simulink model "test_atrias"  (R2014b)
settings: Solver=FixedStepDiscrete  StartTime=0.0  StopTime=inf  FixedStep=0.001  RelTol=1e-3
StartFcn:
  | tg.sampletime = correctedSampleTime;
libraries: xpcethercatlib x62, simulink x41, slrtlib x12
settings Model: xpc_rtwmakecfg_data=_xpcethercatlib_  SimulationMode=external  BufferReuse=off  Creator=drl  LastModifiedBy=drl
settings SolverCC: EnableConcurrentExecution=on  ConcurrentTasks=on
settings OptimizationCC: BlockReduction=off  OptimizeBlockIOStorage=off  BufferReuse=off  GlobalBufferReuse=off  ExpressionFolding=off  LocalBlockOutputs=off
settings HardwareCC: ProdIntDivRoundTo=Zero  ProdEndianess=LittleEndian  ProdLongLongMode=on  ProdHWDeviceType=Generic->32-bit x86 compatible
settings RTWCC: SystemTargetFile=slrt.tlc  TemplateMakefile=slrt_default_tmf  Description=Simulink Real-Time  ProcessScript=slrt_make_rtw_hook  RTWCompilerOptimization=On
settings SimulinkRealTimeCC: GeneratePreprocessorConditionals=Disable all  EnableShiftOperators=on

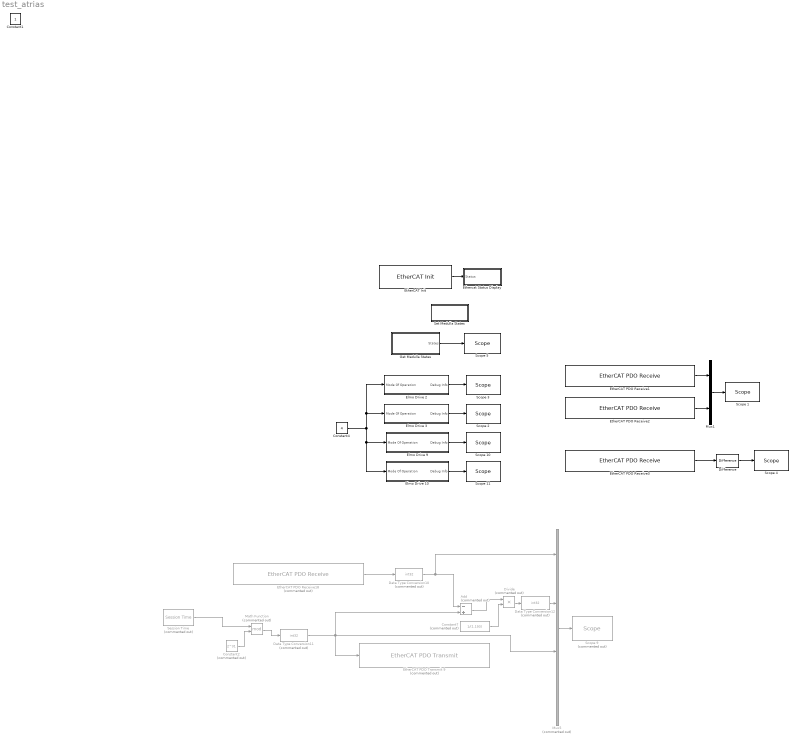
== system test_atrias ==
  Add : Sum  Commented=on  Inputs=-+
  Constant2 : Constant  Commented=on  Value=2^31
  Constant4 : Constant  Value=4  OutDataTypeStr=Inherit: Inherit via back propagation  SampleTime=-1
  Constant7 : Constant  Commented=on  Value=1/(1.193)
  Data Type Conversion10 : DataTypeConversion  Commented=on  OutDataTypeStr=int32
  Data Type Conversion11 : DataTypeConversion  Commented=on  OutDataTypeStr=int32
  Data Type Conversion12 : DataTypeConversion  Commented=on  OutDataTypeStr=int32
  Difference : simulink/Discrete/Difference  ICPrevInput=0.0  InputProcessing=Inherited  OutMin=[]  OutMax=[]  OutDataType=fixdt(1, 16)  OutScaling=2^-10  DoSatur=off
  Divide : Product  Commented=on  Inputs=**
  Elmo Drive 10 : Subsystem
  Elmo Drive 2 : Subsystem
  Elmo Drive 3 : Subsystem
  Elmo Drive 9 : Subsystem
  EtherCAT Init : xpcethercatlib/EtherCAT Init   Priority=0  config_file=8medullas4elmos_eni.xml  device_id=0  pci_bus=2  pci_slot=0  enaDebug=off  enaDC=on  errLink=off  masterDbg=off  stateChgDbg=off  baseClock=off  masterCfg=off  logFile='c:\dbglog.txt'  sample_time=0.001000
  EtherCAT PDO Receive1 : xpcethercatlib/EtherCAT PDO Receive  Priority=2  sig_name=Box 1 (ATRIAS 2.1 Hip (Medulla 1.5)).Hip Encoder.Encoder  sig_offset=504  sig_type=uint32  type_size=32  sig_dim=1  device_id=0  sample_time=0.001000
  EtherCAT PDO Receive18 : xpcethercatlib/EtherCAT PDO Receive  Priority=2  Commented=on  sig_name=Box 6 (ATRIAS 2.1 Leg (Medulla 1.5)).Motor Encoder.Motor Encoder  sig_offset=1648  sig_type=uint32  type_size=32  sig_dim=1  device_id=0  sample_time=0.001000
  EtherCAT PDO Receive2 : xpcethercatlib/EtherCAT PDO Receive  Priority=2  sig_name=Box 12 (ATRIAS 2.1 Boom (Medulla 1.5)).X Encoder.Encoder  sig_offset=2752  sig_type=uint32  type_size=32  sig_dim=1  device_id=0  sample_time=0.001000
  EtherCAT PDO Receive3 : xpcethercatlib/EtherCAT PDO Receive  Priority=2  sig_name=Box 1 (ATRIAS 2.1 Hip (Medulla 1.5)).uController Status.Counter  sig_offset=480  sig_type=uint8  type_size=8  sig_dim=1  device_id=0  sample_time=0.001000
  EtherCAT PDO Transmit 9 : xpcethercatlib/EtherCAT PDO Transmit   Priority=3  Commented=on  sig_name=Box 6 (ATRIAS 2.1 Leg (Medulla 1.5)).uControllerInput.Motor Current  sig_offset=1616  sig_type=int32  type_size=32  sig_dim=1  device_id=0  sample_time=0.001000
  Ethercat Status Display : Subsystem
  Get Medulla States : Subsystem
  Math Function : Math  Commented=on  Operator=mod  SaturateOnIntegerOverflow=on
  Mux1 : Mux  Inputs=2
  Mux5 : Mux  Commented=on
  Scope 1 : slrtlib/Displays and Logging/Scope   scopeno=8  scopetype=Target  autostart=on  viewmode=Graphical sliding  formatstr='%f'  grid=on  ylimits=[0,0]  nosamples=10000  noprepostsamples=0  interleave=1  triggermode=FreeRun  triggersignal=1  trigsignalfromport=off  triggerlevel=0.0  triggerslope=Either  triggerscope=1  triggersample=0  filename=data.dat  mode=Lazy  writesize=512  autorestart=off  dynamicfilemode=off  maxwritefilesize=512*1024^2
  Scope 10 : slrtlib/Displays and Logging/Scope   scopeno=3  scopetype=Target  autostart=on  viewmode=Numerical  formatstr='%f'  grid=on  ylimits=[0,0]  nosamples=10000  noprepostsamples=0  interleave=1  triggermode=FreeRun  triggersignal=1  trigsignalfromport=off  triggerlevel=0.0  triggerslope=Either  triggerscope=1  triggersample=0  filename=data.dat  mode=Lazy  writesize=512  autorestart=off  dynamicfilemode=off  maxwritefilesize=512*1024^2
  Scope 11 : slrtlib/Displays and Logging/Scope   scopeno=4  scopetype=Target  autostart=on  viewmode=Numerical  formatstr='%f'  grid=on  ylimits=[0,0]  nosamples=10000  noprepostsamples=0  interleave=1  triggermode=FreeRun  triggersignal=1  trigsignalfromport=off  triggerlevel=0.0  triggerslope=Either  triggerscope=1  triggersample=0  filename=data.dat  mode=Lazy  writesize=512  autorestart=off  dynamicfilemode=off  maxwritefilesize=512*1024^2
  Scope 2 : slrtlib/Displays and Logging/Scope   scopeno=2  scopetype=Target  autostart=on  viewmode=Numerical  formatstr='%f'  grid=on  ylimits=[0,0]  nosamples=10000  noprepostsamples=0  interleave=1  triggermode=FreeRun  triggersignal=1  trigsignalfromport=off  triggerlevel=0.0  triggerslope=Either  triggerscope=1  triggersample=0  filename=data.dat  mode=Lazy  writesize=512  autorestart=off  dynamicfilemode=off  maxwritefilesize=512*1024^2
  Scope 3 : slrtlib/Displays and Logging/Scope   scopeno=1  scopetype=Target  autostart=on  viewmode=Numerical  formatstr='%f'  grid=on  ylimits=[0,0]  nosamples=10000  noprepostsamples=0  interleave=1  triggermode=FreeRun  triggersignal=1  trigsignalfromport=off  triggerlevel=0.0  triggerslope=Either  triggerscope=1  triggersample=0  filename=data.dat  mode=Lazy  writesize=512  autorestart=off  dynamicfilemode=off  maxwritefilesize=512*1024^2
  Scope 4 : slrtlib/Displays and Logging/Scope   scopeno=9  scopetype=Target  autostart=on  viewmode=Graphical sliding  formatstr='%f'  grid=on  ylimits=[0,0]  nosamples=10000  noprepostsamples=0  interleave=1  triggermode=FreeRun  triggersignal=1  trigsignalfromport=off  triggerlevel=0.0  triggerslope=Either  triggerscope=1  triggersample=0  filename=data.dat  mode=Lazy  writesize=512  autorestart=off  dynamicfilemode=off  maxwritefilesize=512*1024^2
  Scope 5 : slrtlib/Displays and Logging/Scope   scopeno=7  scopetype=Target  autostart=on  viewmode=Numerical  formatstr='%f'  grid=on  ylimits=[0,0]  nosamples=100  noprepostsamples=0  interleave=1  triggermode=FreeRun  triggersignal=1  trigsignalfromport=off  triggerlevel=0.0  triggerslope=Either  triggerscope=1  triggersample=0  filename=data.dat  mode=Lazy  writesize=512  autorestart=off  dynamicfilemode=off  maxwritefilesize=512*1024^2
  Scope 9 : slrtlib/Displays and Logging/Scope   Commented=on  scopeno=10  scopetype=Target  autostart=on  viewmode=Numerical  formatstr='%f'  grid=on  ylimits=[0,0]  nosamples=100  noprepostsamples=0  interleave=1  triggermode=FreeRun  triggersignal=1  trigsignalfromport=off  triggerlevel=0.0  triggerslope=Either  triggerscope=1  triggersample=0  filename=data.dat  mode=Lazy  writesize=512  autorestart=off  dynamicfilemode=off  maxwritefilesize=512*1024^2
  "Session Time " : slrtlib/Target Management/Target Information/Session Time   Commented=on  ts=0.001
  Set Medulla States : Subsystem
  Constant1 : Constant  IOType=siggen
  wires:
  EtherCAT Init/1 -> Ethercat Status Display/1(Status)
  EtherCAT PDO Receive18/1 -> Data Type Conversion10/1
  Mux5/1 -> Scope 9/1
  Data Type Conversion10/1 -> Mux5/1, Add/1
  Constant2/1 -> Math Function/2
  Math Function/1 -> Data Type Conversion11/1
  Data Type Conversion11/1 -> EtherCAT PDO Transmit 9/1, Mux5/3, Add/2
  "Session Time "/1 -> Math Function/1
  Constant7/1 -> Divide/2
  Add/1 -> Divide/1
  Data Type Conversion12/1 -> Mux5/2
  Divide/1 -> Data Type Conversion12/1
  Elmo Drive 3/1(Debug Info) -> Scope 2/1
  Elmo Drive 2/1(Debug Info) -> Scope 3/1
  Elmo Drive 9/1(Debug Info) -> Scope 10/1
  Elmo Drive 10/1(Debug Info) -> Scope 11/1
  Constant4/1 -> Elmo Drive 9/1(Mode Of Operation), Elmo Drive 10/1(Mode Of Operation), Elmo Drive 3/1(Mode Of Operation), Elmo Drive 2/1(Mode Of Operation)
  Get Medulla States/1(States) -> Scope 5/1
  EtherCAT PDO Receive2/1 -> Mux1/2
  EtherCAT PDO Receive1/1 -> Mux1/1
  Mux1/1 -> Scope 1/1
  EtherCAT PDO Receive3/1 -> Difference/1
  Difference/1 -> Scope 4/1

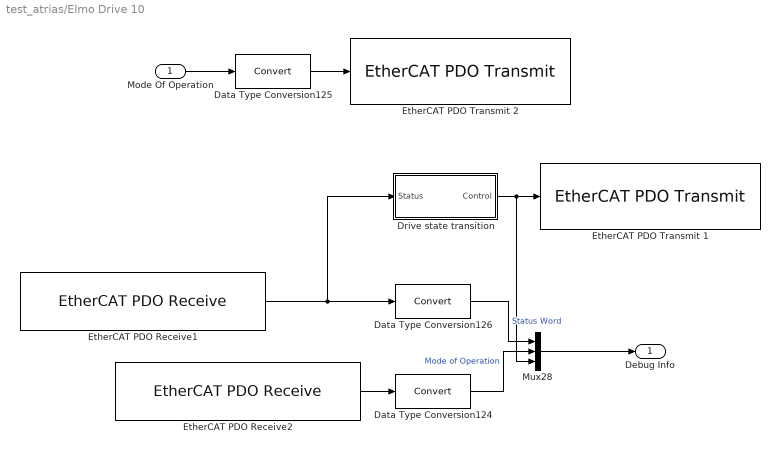
== system test_atrias/Elmo Drive 10 ==
  Mode Of Operation : Inport
  Data Type Conversion124 : DataTypeConversion
  Data Type Conversion125 : DataTypeConversion
  Data Type Conversion126 : DataTypeConversion
  Drive state transition : Subsystem
  EtherCAT PDO Receive1 : xpcethercatlib/EtherCAT PDO Receive  Priority=2  sig_name=Drive 10 (Elmo Drive).Inputs.Status word  sig_offset=3296  sig_type=uint16  type_size=16  sig_dim=1  device_id=0  sample_time=0.001000
  EtherCAT PDO Receive2 : xpcethercatlib/EtherCAT PDO Receive  Priority=2  sig_name=Drive 10 (Elmo Drive).Inputs.Mode of operation display  sig_offset=3312  sig_type=int8  type_size=8  sig_dim=1  device_id=0  sample_time=0.001000
  EtherCAT PDO Transmit 1 : xpcethercatlib/EtherCAT PDO Transmit   Priority=3  sig_name=Drive 10 (Elmo Drive).Outputs.Control word  sig_offset=3264  sig_type=uint16  type_size=16  sig_dim=1  device_id=0  sample_time=0.001000
  EtherCAT PDO Transmit 2 : xpcethercatlib/EtherCAT PDO Transmit   Priority=3  sig_name=Drive 10 (Elmo Drive).Outputs.Mode of operation  sig_offset=3280  sig_type=int8  type_size=8  sig_dim=1  device_id=0  sample_time=0.001000
  Mux28 : Mux  Inputs=3
  Debug Info : Outport
  wires:
  EtherCAT PDO Receive1/1 -> Drive state transition/1(Status), Data Type Conversion126/1
  EtherCAT PDO Receive2/1 -> Data Type Conversion124/1
  Mux28/1 -> Debug Info/1
  Data Type Conversion126/1 -> Mux28/1  "Status Word"
  Data Type Conversion124/1 -> Mux28/2  "Mode of Operation"
  Mode Of Operation/1 -> Data Type Conversion125/1
  Drive state transition/1(Control) -> Mux28/3, EtherCAT PDO Transmit 1/1
  Data Type Conversion125/1 -> EtherCAT PDO Transmit 2/1

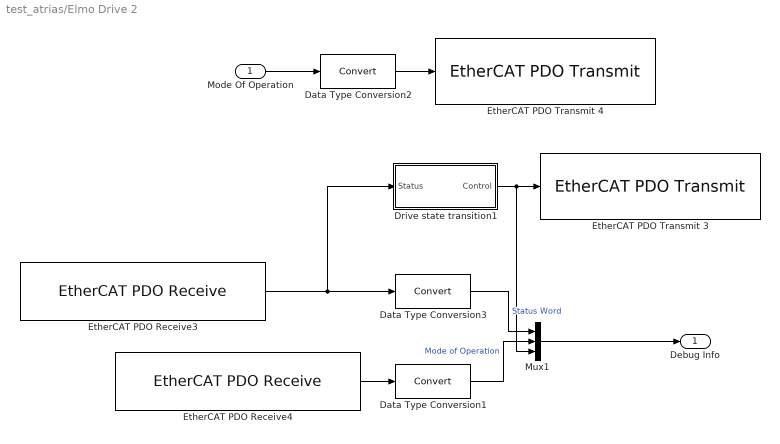
== system test_atrias/Elmo Drive 2 ==
  Mode Of Operation : Inport
  Data Type Conversion1 : DataTypeConversion
  Data Type Conversion2 : DataTypeConversion
  Data Type Conversion3 : DataTypeConversion
  Drive state transition1 : Subsystem
  EtherCAT PDO Receive3 : xpcethercatlib/EtherCAT PDO Receive  Priority=2  sig_name=Drive 2 (Elmo Drive).Inputs.Status word  sig_offset=3056  sig_type=uint16  type_size=16  sig_dim=1  device_id=0  sample_time=0.001000
  EtherCAT PDO Receive4 : xpcethercatlib/EtherCAT PDO Receive  Priority=2  sig_name=Drive 2 (Elmo Drive).Inputs.Mode of operation display  sig_offset=3072  sig_type=int8  type_size=8  sig_dim=1  device_id=0  sample_time=0.001000
  EtherCAT PDO Transmit 3 : xpcethercatlib/EtherCAT PDO Transmit   Priority=3  sig_name=Drive 2 (Elmo Drive).Outputs.Control word  sig_offset=3024  sig_type=uint16  type_size=16  sig_dim=1  device_id=0  sample_time=0.001000
  EtherCAT PDO Transmit 4 : xpcethercatlib/EtherCAT PDO Transmit   Priority=3  sig_name=Drive 2 (Elmo Drive).Outputs.Mode of operation  sig_offset=3040  sig_type=int8  type_size=8  sig_dim=1  device_id=0  sample_time=0.001000
  Mux1 : Mux  Inputs=3
  Debug Info : Outport
  wires:
  EtherCAT PDO Receive3/1 -> Drive state transition1/1(Status), Data Type Conversion3/1
  EtherCAT PDO Receive4/1 -> Data Type Conversion1/1
  Mux1/1 -> Debug Info/1
  Data Type Conversion3/1 -> Mux1/1  "Status Word"
  Data Type Conversion1/1 -> Mux1/2  "Mode of Operation"
  Mode Of Operation/1 -> Data Type Conversion2/1
  Drive state transition1/1(Control) -> Mux1/3, EtherCAT PDO Transmit 3/1
  Data Type Conversion2/1 -> EtherCAT PDO Transmit 4/1

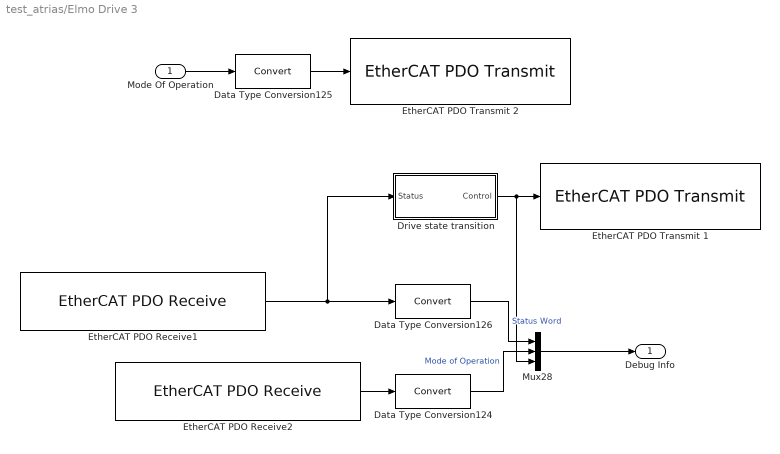
== system test_atrias/Elmo Drive 3 ==
  Mode Of Operation : Inport
  Data Type Conversion124 : DataTypeConversion
  Data Type Conversion125 : DataTypeConversion
  Data Type Conversion126 : DataTypeConversion
  Drive state transition : Subsystem
  EtherCAT PDO Receive1 : xpcethercatlib/EtherCAT PDO Receive  Priority=2  sig_name=Drive 3 (Elmo Drive).Inputs.Status word  sig_offset=3136  sig_type=uint16  type_size=16  sig_dim=1  device_id=0  sample_time=0.001000
  EtherCAT PDO Receive2 : xpcethercatlib/EtherCAT PDO Receive  Priority=2  sig_name=Drive 3 (Elmo Drive).Inputs.Mode of operation display  sig_offset=3152  sig_type=int8  type_size=8  sig_dim=1  device_id=0  sample_time=0.001000
  EtherCAT PDO Transmit 1 : xpcethercatlib/EtherCAT PDO Transmit   Priority=3  sig_name=Drive 3 (Elmo Drive).Outputs.Control word  sig_offset=3104  sig_type=uint16  type_size=16  sig_dim=1  device_id=0  sample_time=0.001000
  EtherCAT PDO Transmit 2 : xpcethercatlib/EtherCAT PDO Transmit   Priority=3  sig_name=Drive 3 (Elmo Drive).Outputs.Mode of operation  sig_offset=3120  sig_type=int8  type_size=8  sig_dim=1  device_id=0  sample_time=0.001000
  Mux28 : Mux  Inputs=3
  Debug Info : Outport
  wires:
  EtherCAT PDO Receive1/1 -> Drive state transition/1(Status), Data Type Conversion126/1
  EtherCAT PDO Receive2/1 -> Data Type Conversion124/1
  Mux28/1 -> Debug Info/1
  Data Type Conversion126/1 -> Mux28/1  "Status Word"
  Data Type Conversion124/1 -> Mux28/2  "Mode of Operation"
  Mode Of Operation/1 -> Data Type Conversion125/1
  Drive state transition/1(Control) -> Mux28/3, EtherCAT PDO Transmit 1/1
  Data Type Conversion125/1 -> EtherCAT PDO Transmit 2/1

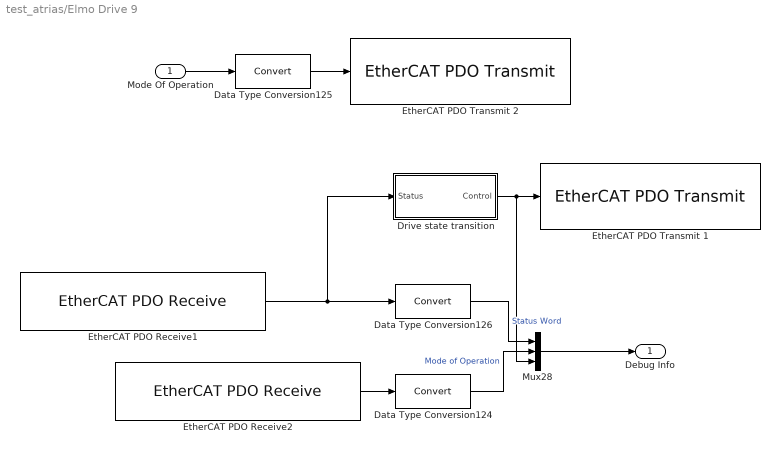
== system test_atrias/Elmo Drive 9 ==
  Mode Of Operation : Inport
  Data Type Conversion124 : DataTypeConversion
  Data Type Conversion125 : DataTypeConversion
  Data Type Conversion126 : DataTypeConversion
  Drive state transition : Subsystem
  EtherCAT PDO Receive1 : xpcethercatlib/EtherCAT PDO Receive  Priority=2  sig_name=Drive 9 (Elmo Drive).Inputs.Status word  sig_offset=3216  sig_type=uint16  type_size=16  sig_dim=1  device_id=0  sample_time=0.001000
  EtherCAT PDO Receive2 : xpcethercatlib/EtherCAT PDO Receive  Priority=2  sig_name=Drive 9 (Elmo Drive).Inputs.Mode of operation display  sig_offset=3232  sig_type=int8  type_size=8  sig_dim=1  device_id=0  sample_time=0.001000
  EtherCAT PDO Transmit 1 : xpcethercatlib/EtherCAT PDO Transmit   Priority=3  sig_name=Drive 9 (Elmo Drive).Outputs.Control word  sig_offset=3184  sig_type=uint16  type_size=16  sig_dim=1  device_id=0  sample_time=0.001000
  EtherCAT PDO Transmit 2 : xpcethercatlib/EtherCAT PDO Transmit   Priority=3  sig_name=Drive 9 (Elmo Drive).Outputs.Mode of operation  sig_offset=3200  sig_type=int8  type_size=8  sig_dim=1  device_id=0  sample_time=0.001000
  Mux28 : Mux  Inputs=3
  Debug Info : Outport
  wires:
  Data Type Conversion125/1 -> EtherCAT PDO Transmit 2/1
  Drive state transition/1(Control) -> EtherCAT PDO Transmit 1/1, Mux28/3
  Mode Of Operation/1 -> Data Type Conversion125/1
  Data Type Conversion124/1 -> Mux28/2  "Mode of Operation"
  Data Type Conversion126/1 -> Mux28/1  "Status Word"
  Mux28/1 -> Debug Info/1
  EtherCAT PDO Receive2/1 -> Data Type Conversion124/1
  EtherCAT PDO Receive1/1 -> Data Type Conversion126/1, Drive state transition/1(Status)

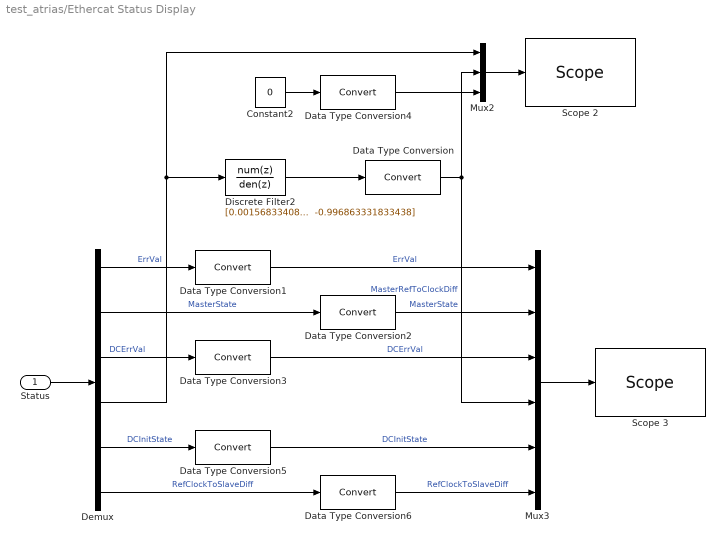
== system test_atrias/Ethercat Status Display ==
  Status : Inport
  Constant2 : Constant  Value=0  OutDataTypeStr=Inherit: Inherit via back propagation  SampleTime=-1
  Data Type Conversion{,1..6} (7 alike) : DataTypeConversion
  Demux : Demux  Outputs=6
  Discrete Filter2 : DiscreteFilter  Numerator="[0.001568334083281   0.001568334083281]"  Denominator="[1.000000000000000  -0.996863331833438]"  a0EqualsOne=on
  Mux2 : Mux  Inputs=3
  Mux3 : Mux  Inputs=6
  Scope 2 : slrtlib/Displays and Logging/Scope   scopeno=5  scopetype=Target  autostart=on  viewmode=Graphical rolling  formatstr='%f'  grid=on  ylimits=[0,0]  nosamples=10000  noprepostsamples=0  interleave=1  triggermode=FreeRun  triggersignal=1  trigsignalfromport=off  triggerlevel=0.0  triggerslope=Either  triggerscope=1  triggersample=0  filename=data.dat  mode=Lazy  writesize=512  autorestart=off  dynamicfilemode=off  maxwritefilesize=512*1024^2
  Scope 3 : slrtlib/Displays and Logging/Scope   scopeno=6  scopetype=Target  autostart=on  viewmode=Numerical  formatstr='%15.6f'  grid=on  ylimits=[0,0]  nosamples=100  noprepostsamples=0  interleave=1  triggermode=FreeRun  triggersignal=1  trigsignalfromport=off  triggerlevel=0.0  triggerslope=Either  triggerscope=1  triggersample=0  filename=data.dat  mode=Lazy  writesize=512  autorestart=off  dynamicfilemode=off  maxwritefilesize=512*1024^2
  wires:
  Status/1 -> Demux/1
  Demux/4 -> Discrete Filter2/1, Mux2/1
  Discrete Filter2/1 -> Data Type Conversion/1
  Mux2/1 -> Scope 2/1
  Constant2/1 -> Data Type Conversion4/1
  Data Type Conversion4/1 -> Mux2/3
  Mux3/1 -> Scope 3/1
  Data Type Conversion/1 -> Mux3/4, Mux2/2  "MasterRefToClockDiff"
  Data Type Conversion1/1 -> Mux3/1  "ErrVal"
  Data Type Conversion2/1 -> Mux3/2  "MasterState"
  Data Type Conversion3/1 -> Mux3/3  "DCErrVal"
  Data Type Conversion5/1 -> Mux3/5  "DCInitState"
  Data Type Conversion6/1 -> Mux3/6  "RefClockToSlaveDiff"
  Demux/1 -> Data Type Conversion1/1  "ErrVal"
  Demux/2 -> Data Type Conversion2/1  "MasterState"
  Demux/3 -> Data Type Conversion3/1  "DCErrVal"
  Demux/5 -> Data Type Conversion5/1  "DCInitState"
  Demux/6 -> Data Type Conversion6/1  "RefClockToSlaveDiff"

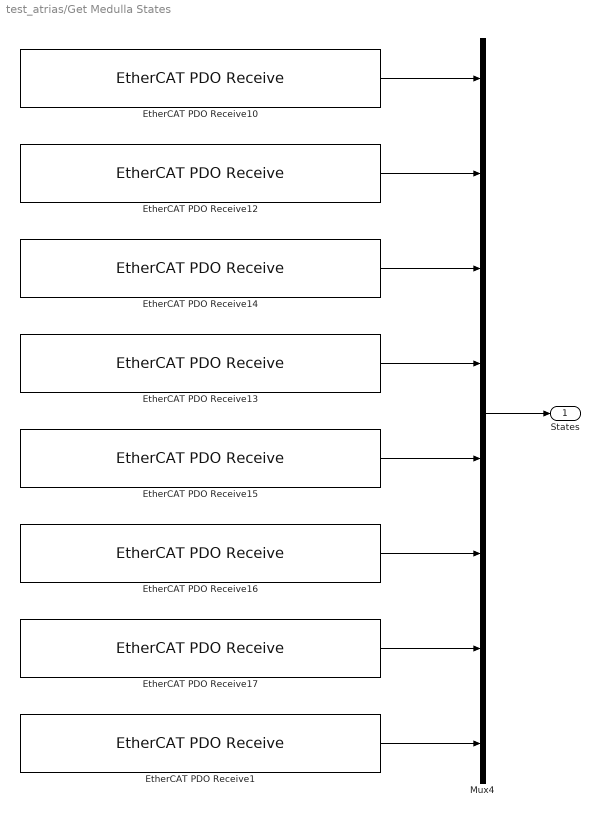
== system test_atrias/Get Medulla States ==
  EtherCAT PDO Receive1 : xpcethercatlib/EtherCAT PDO Receive  Priority=2  sig_name=Box 12 (ATRIAS 2.1 Boom (Medulla 1.5)).uController Status.State  sig_offset=2728  sig_type=uint8  type_size=8  sig_dim=1  device_id=0  sample_time=0.001000
  EtherCAT PDO Receive10 : xpcethercatlib/EtherCAT PDO Receive  Priority=2  sig_name=Box 1 (ATRIAS 2.1 Hip (Medulla 1.5)).uController Status.State  sig_offset=472  sig_type=uint8  type_size=8  sig_dim=1  device_id=0  sample_time=0.001000
  EtherCAT PDO Receive12 : xpcethercatlib/EtherCAT PDO Receive  Priority=2  sig_name=Box 4 (ATRIAS 2.1 IMU (Medulla 1.5)).uController Status.State  sig_offset=720  sig_type=uint8  type_size=8  sig_dim=1  device_id=0  sample_time=0.001000
  EtherCAT PDO Receive13 : xpcethercatlib/EtherCAT PDO Receive  Priority=2  sig_name=Box 6 (ATRIAS 2.1 Leg (Medulla 1.5)).uController Status.State  sig_offset=1352  sig_type=uint8  type_size=8  sig_dim=1  device_id=0  sample_time=0.001000
  EtherCAT PDO Receive14 : xpcethercatlib/EtherCAT PDO Receive  Priority=2  sig_name=Box 5 (ATRIAS 2.1 Leg (Medulla 1.5)).uController Status.State  sig_offset=976  sig_type=uint8  type_size=8  sig_dim=1  device_id=0  sample_time=0.001000
  EtherCAT PDO Receive15 : xpcethercatlib/EtherCAT PDO Receive  Priority=2  sig_name=Box 7 (ATRIAS 2.1 Leg (Medulla 1.5)).uController Status.State  sig_offset=1728  sig_type=uint8  type_size=8  sig_dim=1  device_id=0  sample_time=0.001000
  EtherCAT PDO Receive16 : xpcethercatlib/EtherCAT PDO Receive  Priority=2  sig_name=Box 8 (ATRIAS 2.1 Leg (Medulla 1.5)).uController Status.State  sig_offset=2104  sig_type=uint8  type_size=8  sig_dim=1  device_id=0  sample_time=0.001000
  EtherCAT PDO Receive17 : xpcethercatlib/EtherCAT PDO Receive  Priority=2  sig_name=Box 11 (ATRIAS 2.1 Hip (Medulla 1.5)).uController Status.State  sig_offset=2480  sig_type=uint8  type_size=8  sig_dim=1  device_id=0  sample_time=0.001000
  Mux4 : Mux  Inputs=8
  States : Outport
  wires:
  EtherCAT PDO Receive1/1 -> Mux4/8
  EtherCAT PDO Receive10/1 -> Mux4/1
  EtherCAT PDO Receive12/1 -> Mux4/2
  EtherCAT PDO Receive14/1 -> Mux4/3
  Mux4/1 -> States/1
  EtherCAT PDO Receive13/1 -> Mux4/4
  EtherCAT PDO Receive15/1 -> Mux4/5
  EtherCAT PDO Receive16/1 -> Mux4/6
  EtherCAT PDO Receive17/1 -> Mux4/7

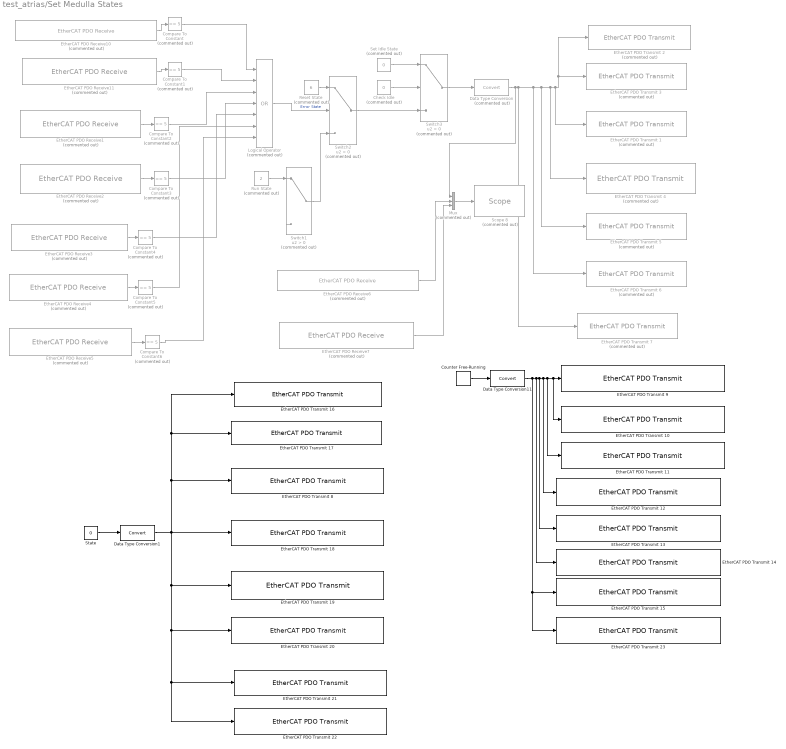
== system test_atrias/Set Medulla States ==
  Check Idle : Constant  Commented=on  Value=0
  Compare To Constant{,1..6} (7 alike) : simulink/Logic and Bit Operations/Compare To Constant  Commented=on  relop===  const=5  OutDataTypeStr=boolean
  Counter Free-Running : simulink/Sources/Counter Free-Running  NumBits=16  tsamp=-1
  Data Type Conversion : DataTypeConversion  Commented=on
  Data Type Conversion1 : DataTypeConversion
  Data Type Conversion11 : DataTypeConversion
  EtherCAT PDO Receive1 : xpcethercatlib/EtherCAT PDO Receive  Priority=2  Commented=on  sig_name=Box 5 (ATRIAS 2.1 Leg (Medulla 1.5)).uController Status.State  sig_offset=1224  sig_type=uint8  type_size=8  sig_dim=1  device_id=0  sample_time=0.001000
  EtherCAT PDO Receive10 : xpcethercatlib/EtherCAT PDO Receive  Priority=2  Commented=on  sig_name=Box 1 (ATRIAS 2.1 Hip (Medulla 1.5)).uController Status.State  sig_offset=600  sig_type=uint8  type_size=8  sig_dim=1  device_id=0  sample_time=0.001000
  EtherCAT PDO Receive11 : xpcethercatlib/EtherCAT PDO Receive  Priority=2  Commented=on  sig_name=Box 4 (ATRIAS 2.1 Leg (Medulla 1.5)).uController Status.State  sig_offset=848  sig_type=uint8  type_size=8  sig_dim=1  device_id=0  sample_time=0.001000
  EtherCAT PDO Receive2 : xpcethercatlib/EtherCAT PDO Receive  Priority=2  Commented=on  sig_name=Box 6 (ATRIAS 2.1 Leg (Medulla 1.5)).uController Status.State  sig_offset=1600  sig_type=uint8  type_size=8  sig_dim=1  device_id=0  sample_time=0.001000
  EtherCAT PDO Receive3 : xpcethercatlib/EtherCAT PDO Receive  Priority=2  Commented=on  sig_name=Box 7 (ATRIAS 2.1 Leg (Medulla 1.5)).uController Status.State  sig_offset=1976  sig_type=uint8  type_size=8  sig_dim=1  device_id=0  sample_time=0.001000
  EtherCAT PDO Receive4 : xpcethercatlib/EtherCAT PDO Receive  Priority=2  Commented=on  sig_name=Box 10 (ATRIAS 2.1 Hip (Medulla 1.5)).uController Status.State  sig_offset=2352  sig_type=uint8  type_size=8  sig_dim=1  device_id=0  sample_time=0.001000
  EtherCAT PDO Receive5 : xpcethercatlib/EtherCAT PDO Receive  Priority=2  Commented=on  sig_name=Box 11 (ATRIAS 2.1 Boom (Medulla 1.5)).uController Status.State  sig_offset=2600  sig_type=uint8  type_size=8  sig_dim=1  device_id=0  sample_time=0.001000
  EtherCAT PDO Receive6 : xpcethercatlib/EtherCAT PDO Receive  Priority=2  Commented=on  sig_name=Box 1 (ATRIAS 2.1 Hip (Medulla 1.5)).uController Status.Error Flags  sig_offset=616  sig_type=uint8  type_size=8  sig_dim=1  device_id=0  sample_time=0.001000
  EtherCAT PDO Receive7 : xpcethercatlib/EtherCAT PDO Receive  Priority=2  Commented=on  sig_name=Box 4 (ATRIAS 2.1 Leg (Medulla 1.5)).uController Status.Error Flags  sig_offset=864  sig_type=uint8  type_size=8  sig_dim=1  device_id=0  sample_time=0.001000
  EtherCAT PDO Transmit 1 : xpcethercatlib/EtherCAT PDO Transmit   Priority=3  Commented=on  sig_name=Box 5 (ATRIAS 2.1 Leg (Medulla 1.5)).uControllerInput.Command  sig_offset=1216  sig_type=uint8  type_size=8  sig_dim=1  device_id=0  sample_time=0.001000
  EtherCAT PDO Transmit 10 : xpcethercatlib/EtherCAT PDO Transmit   Priority=3  sig_name=Box 4 (ATRIAS 2.1 IMU (Medulla 1.5)).uControllerInput.Counter  sig_offset=720  sig_type=uint16  type_size=16  sig_dim=1  device_id=0  sample_time=0.001000
  EtherCAT PDO Transmit 11 : xpcethercatlib/EtherCAT PDO Transmit   Priority=3  sig_name=Box 5 (ATRIAS 2.1 Leg (Medulla 1.5)).uControllerInput.Counter  sig_offset=976  sig_type=uint16  type_size=16  sig_dim=1  device_id=0  sample_time=0.001000
  EtherCAT PDO Transmit 12 : xpcethercatlib/EtherCAT PDO Transmit   Priority=3  sig_name=Box 6 (ATRIAS 2.1 Leg (Medulla 1.5)).uControllerInput.Counter  sig_offset=1352  sig_type=uint16  type_size=16  sig_dim=1  device_id=0  sample_time=0.001000
  EtherCAT PDO Transmit 13 : xpcethercatlib/EtherCAT PDO Transmit   Priority=3  sig_name=Box 7 (ATRIAS 2.1 Leg (Medulla 1.5)).uControllerInput.Counter  sig_offset=1728  sig_type=uint16  type_size=16  sig_dim=1  device_id=0  sample_time=0.001000
  EtherCAT PDO Transmit 14 : xpcethercatlib/EtherCAT PDO Transmit   Priority=3  sig_name=Box 8 (ATRIAS 2.1 Leg (Medulla 1.5)).uControllerInput.Counter  sig_offset=2104  sig_type=uint16  type_size=16  sig_dim=1  device_id=0  sample_time=0.001000
  EtherCAT PDO Transmit 15 : xpcethercatlib/EtherCAT PDO Transmit   Priority=3  sig_name=Box 11 (ATRIAS 2.1 Hip (Medulla 1.5)).uControllerInput.Counter  sig_offset=2480  sig_type=uint16  type_size=16  sig_dim=1  device_id=0  sample_time=0.001000
  EtherCAT PDO Transmit 16 : xpcethercatlib/EtherCAT PDO Transmit   Priority=3  sig_name=Box 1 (ATRIAS 2.1 Hip (Medulla 1.5)).uControllerInput.Command  sig_offset=464  sig_type=uint8  type_size=8  sig_dim=1  device_id=0  sample_time=0.001000
  EtherCAT PDO Transmit 17 : xpcethercatlib/EtherCAT PDO Transmit   Priority=3  sig_name=Box 4 (ATRIAS 2.1 IMU (Medulla 1.5)).uControllerInput.Command  sig_offset=712  sig_type=uint8  type_size=8  sig_dim=1  device_id=0  sample_time=0.001000
  EtherCAT PDO Transmit 18 : xpcethercatlib/EtherCAT PDO Transmit   Priority=3  sig_name=Box 6 (ATRIAS 2.1 Leg (Medulla 1.5)).uControllerInput.Command  sig_offset=1344  sig_type=uint8  type_size=8  sig_dim=1  device_id=0  sample_time=0.001000
  EtherCAT PDO Transmit 19 : xpcethercatlib/EtherCAT PDO Transmit   Priority=3  sig_name=Box 7 (ATRIAS 2.1 Leg (Medulla 1.5)).uControllerInput.Command  sig_offset=1720  sig_type=uint8  type_size=8  sig_dim=1  device_id=0  sample_time=0.001000
  EtherCAT PDO Transmit 2 : xpcethercatlib/EtherCAT PDO Transmit   Priority=3  Commented=on  sig_name=Box 1 (ATRIAS 2.1 Hip (Medulla 1.5)).uControllerInput.Command  sig_offset=592  sig_type=uint8  type_size=8  sig_dim=1  device_id=0  sample_time=0.001000
  EtherCAT PDO Transmit 20 : xpcethercatlib/EtherCAT PDO Transmit   Priority=3  sig_name=Box 8 (ATRIAS 2.1 Leg (Medulla 1.5)).uControllerInput.Command  sig_offset=2096  sig_type=uint8  type_size=8  sig_dim=1  device_id=0  sample_time=0.001000
  EtherCAT PDO Transmit 21 : xpcethercatlib/EtherCAT PDO Transmit   Priority=3  sig_name=Box 11 (ATRIAS 2.1 Hip (Medulla 1.5)).uControllerInput.Command  sig_offset=2472  sig_type=uint8  type_size=8  sig_dim=1  device_id=0  sample_time=0.001000
  EtherCAT PDO Transmit 22 : xpcethercatlib/EtherCAT PDO Transmit   Priority=3  sig_name=Box 12 (ATRIAS 2.1 Boom (Medulla 1.5)).uControllerInput.Command  sig_offset=2720  sig_type=uint8  type_size=8  sig_dim=1  device_id=0  sample_time=0.001000
  EtherCAT PDO Transmit 23 : xpcethercatlib/EtherCAT PDO Transmit   Priority=3  sig_name=Box 12 (ATRIAS 2.1 Boom (Medulla 1.5)).uControllerInput.Counter  sig_offset=2728  sig_type=uint16  type_size=16  sig_dim=1  device_id=0  sample_time=0.001000
  EtherCAT PDO Transmit 3 : xpcethercatlib/EtherCAT PDO Transmit   Priority=3  Commented=on  sig_name=Box 4 (ATRIAS 2.1 Leg (Medulla 1.5)).uControllerInput.Command  sig_offset=840  sig_type=uint8  type_size=8  sig_dim=1  device_id=0  sample_time=0.001000
  EtherCAT PDO Transmit 4 : xpcethercatlib/EtherCAT PDO Transmit   Priority=3  Commented=on  sig_name=Box 6 (ATRIAS 2.1 Leg (Medulla 1.5)).uControllerInput.Command  sig_offset=1592  sig_type=uint8  type_size=8  sig_dim=1  device_id=0  sample_time=0.001000
  EtherCAT PDO Transmit 5 : xpcethercatlib/EtherCAT PDO Transmit   Priority=3  Commented=on  sig_name=Box 7 (ATRIAS 2.1 Leg (Medulla 1.5)).uControllerInput.Command  sig_offset=1968  sig_type=uint8  type_size=8  sig_dim=1  device_id=0  sample_time=0.001000
  EtherCAT PDO Transmit 6 : xpcethercatlib/EtherCAT PDO Transmit   Priority=3  Commented=on  sig_name=Box 10 (ATRIAS 2.1 Hip (Medulla 1.5)).uControllerInput.Command  sig_offset=2344  sig_type=uint8  type_size=8  sig_dim=1  device_id=0  sample_time=0.001000
  EtherCAT PDO Transmit 7 : xpcethercatlib/EtherCAT PDO Transmit   Priority=3  Commented=on  sig_name=Box 11 (ATRIAS 2.1 Boom (Medulla 1.5)).uControllerInput.Command  sig_offset=2592  sig_type=uint8  type_size=8  sig_dim=1  device_id=0  sample_time=0.001000
  EtherCAT PDO Transmit 8 : xpcethercatlib/EtherCAT PDO Transmit   Priority=3  sig_name=Box 5 (ATRIAS 2.1 Leg (Medulla 1.5)).uControllerInput.Command  sig_offset=968  sig_type=uint8  type_size=8  sig_dim=1  device_id=0  sample_time=0.001000
  EtherCAT PDO Transmit 9 : xpcethercatlib/EtherCAT PDO Transmit   Priority=3  sig_name=Box 1 (ATRIAS 2.1 Hip (Medulla 1.5)).uControllerInput.Counter  sig_offset=472  sig_type=uint16  type_size=16  sig_dim=1  device_id=0  sample_time=0.001000
  Logical Operator : Logic  Commented=on  Operator=OR  Inputs=7  AllPortsSameDT=off  OutDataTypeStr=boolean
  Mux : Mux  Commented=on  Inputs=3
  Reset State : Constant  Commented=on  Value=6
  Run State : Constant  Commented=on  Value=2
  Scope 8 : slrtlib/Displays and Logging/Scope   Commented=on  scopeno=10  scopetype=Target  autostart=on  viewmode=Numerical  formatstr='%f'  grid=on  ylimits=[0,0]  nosamples=100  noprepostsamples=0  interleave=1  triggermode=FreeRun  triggersignal=1  trigsignalfromport=off  triggerlevel=0.0  triggerslope=Either  triggerscope=1  triggersample=0  filename=data.dat  mode=Lazy  writesize=512  autorestart=off  dynamicfilemode=off  maxwritefilesize=512*1024^2
  Set Idle State : Constant  Commented=on  Value=0
  State : Constant  Value=0
  Switch1 : Switch  Commented=on  Criteria=u2 > Threshold
  Switch2 : Switch  Commented=on  Criteria=u2 > Threshold
  Switch3 : Switch  Commented=on  Criteria=u2 > Threshold
  wires:
  Run State/1 -> Switch1/1
  Compare To Constant1/1 -> Logical Operator/2
  Compare To Constant/1 -> Logical Operator/1
  EtherCAT PDO Receive10/1 -> Compare To Constant/1
  EtherCAT PDO Receive11/1 -> Compare To Constant1/1
  Logical Operator/1 -> Switch2/2  "Error State"
  Switch1/1 -> Switch2/3
  Reset State/1 -> Switch2/1
  Switch2/1 -> Switch3/3
  Data Type Conversion/1 -> Mux/1, EtherCAT PDO Transmit 7/1, EtherCAT PDO Transmit 6/1, EtherCAT PDO Transmit 5/1, EtherCAT PDO Transmit 4/1, EtherCAT PDO Transmit 1/1, EtherCAT PDO Transmit 2/1, EtherCAT PDO Transmit 3/1
  Set Idle State/1 -> Switch3/1
  Switch3/1 -> Data Type Conversion/1
  Check Idle/1 -> Switch3/2
  Data Type Conversion11/1 -> EtherCAT PDO Transmit 23/1, EtherCAT PDO Transmit 15/1, EtherCAT PDO Transmit 14/1, EtherCAT PDO Transmit 13/1, EtherCAT PDO Transmit 12/1, EtherCAT PDO Transmit 11/1, EtherCAT PDO Transmit 10/1, EtherCAT PDO Transmit 9/1
  Counter Free-Running/1 -> Data Type Conversion11/1
  Compare To Constant2/1 -> Logical Operator/3
  Compare To Constant3/1 -> Logical Operator/4
  Compare To Constant4/1 -> Logical Operator/5
  Compare To Constant5/1 -> Logical Operator/6
  Compare To Constant6/1 -> Logical Operator/7
  EtherCAT PDO Receive1/1 -> Compare To Constant2/1
  EtherCAT PDO Receive2/1 -> Compare To Constant3/1
  EtherCAT PDO Receive3/1 -> Compare To Constant4/1
  EtherCAT PDO Receive4/1 -> Compare To Constant5/1
  EtherCAT PDO Receive5/1 -> Compare To Constant6/1
  Mux/1 -> Scope 8/1
  EtherCAT PDO Receive6/1 -> Mux/2
  EtherCAT PDO Receive7/1 -> Mux/3
  State/1 -> Data Type Conversion1/1
  Data Type Conversion1/1 -> EtherCAT PDO Transmit 17/1, EtherCAT PDO Transmit 16/1, EtherCAT PDO Transmit 8/1, EtherCAT PDO Transmit 19/1, EtherCAT PDO Transmit 20/1, EtherCAT PDO Transmit 22/1, EtherCAT PDO Transmit 21/1, EtherCAT PDO Transmit 18/1

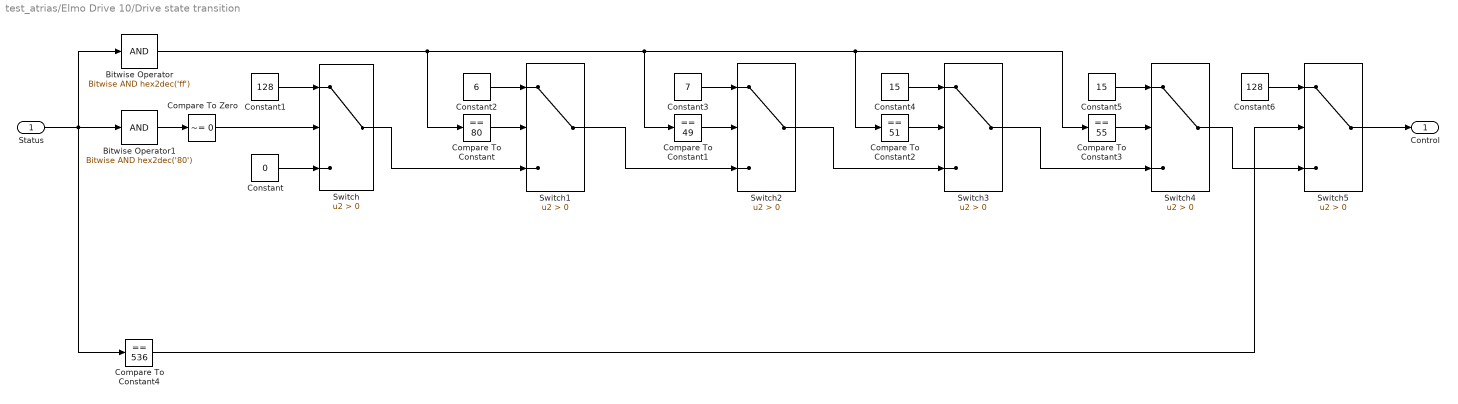
== system test_atrias/Elmo Drive 10/Drive state transition ==
  Status : Inport
  Bitwise Operator : simulink/Logic and Bit Operations/Bitwise Operator  logicop=AND  UseBitMask=on  BitMask=hex2dec('ff')  BitMaskRealWorld=Stored Integer
  Bitwise Operator1 : simulink/Logic and Bit Operations/Bitwise Operator  logicop=AND  UseBitMask=on  BitMask=hex2dec('80')  BitMaskRealWorld=Stored Integer
  Compare To Constant : simulink/Logic and Bit Operations/Compare To Constant  relop===  const=80  OutDataTypeStr=boolean
  Compare To Constant1 : simulink/Logic and Bit Operations/Compare To Constant  relop===  const=49  OutDataTypeStr=boolean
  Compare To Constant2 : simulink/Logic and Bit Operations/Compare To Constant  relop===  const=51  OutDataTypeStr=boolean
  Compare To Constant3 : simulink/Logic and Bit Operations/Compare To Constant  relop===  const=55  OutDataTypeStr=boolean
  Compare To Constant4 : simulink/Logic and Bit Operations/Compare To Constant  relop===  const=536  OutDataTypeStr=boolean
  Compare To Zero : simulink/Logic and Bit Operations/Compare To Zero  relop=~=  OutDataTypeStr=boolean
  Constant : Constant  Value=0  OutDataTypeStr=uint16
  Constant1 : Constant  Value=128  OutDataTypeStr=uint16
  Constant2 : Constant  Value=6  OutDataTypeStr=uint16
  Constant3 : Constant  Value=7  OutDataTypeStr=uint16
  Constant4 : Constant  Value=15  OutDataTypeStr=uint16
  Constant5 : Constant  Value=15  OutDataTypeStr=uint16
  Constant6 : Constant  Value=128  OutDataTypeStr=uint16
  Switch{,1..5} (6 alike) : Switch  Criteria=u2 > Threshold
  Control : Outport
  wires:
  Status/1 -> Compare To Constant4/1, Bitwise Operator/1, Bitwise Operator1/1
  Bitwise Operator1/1 -> Compare To Zero/1
  Compare To Zero/1 -> Switch/2
  Constant1/1 -> Switch/1
  Constant/1 -> Switch/3
  Compare To Constant/1 -> Switch1/2
  Switch/1 -> Switch1/3
  Bitwise Operator/1 -> Compare To Constant3/1, Compare To Constant2/1, Compare To Constant1/1, Compare To Constant/1
  Constant2/1 -> Switch1/1
  Compare To Constant1/1 -> Switch2/2
  Switch1/1 -> Switch2/3
  Constant3/1 -> Switch2/1
  Compare To Constant2/1 -> Switch3/2
  Switch2/1 -> Switch3/3
  Constant4/1 -> Switch3/1
  Compare To Constant3/1 -> Switch4/2
  Switch3/1 -> Switch4/3
  Constant5/1 -> Switch4/1
  Switch4/1 -> Switch5/3
  Compare To Constant4/1 -> Switch5/2
  Switch5/1 -> Control/1
  Constant6/1 -> Switch5/1

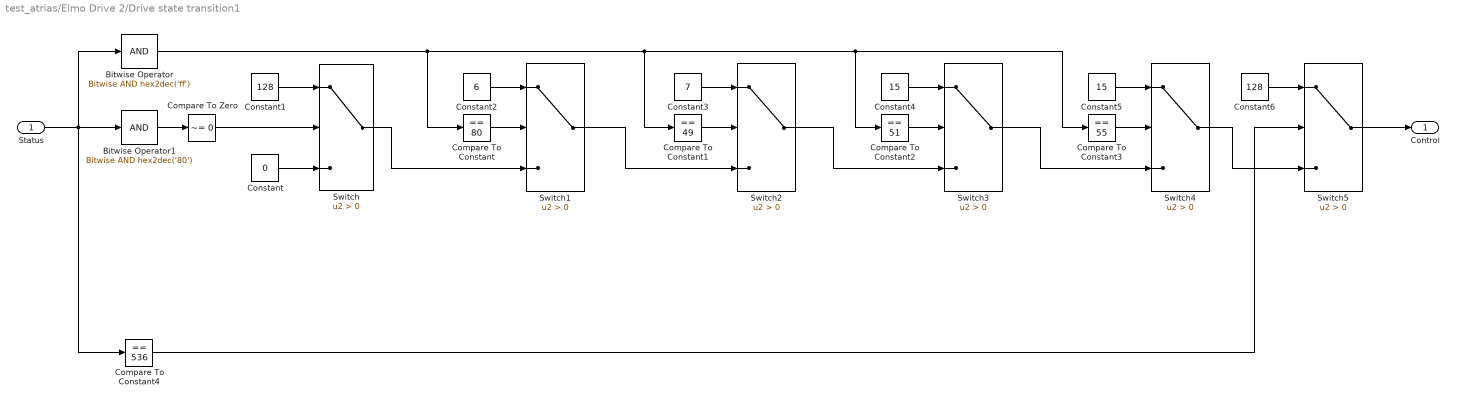
== system test_atrias/Elmo Drive 2/Drive state transition1 ==
  Status : Inport
  Bitwise Operator : simulink/Logic and Bit Operations/Bitwise Operator  logicop=AND  UseBitMask=on  BitMask=hex2dec('ff')  BitMaskRealWorld=Stored Integer
  Bitwise Operator1 : simulink/Logic and Bit Operations/Bitwise Operator  logicop=AND  UseBitMask=on  BitMask=hex2dec('80')  BitMaskRealWorld=Stored Integer
  Compare To Constant : simulink/Logic and Bit Operations/Compare To Constant  relop===  const=80  OutDataTypeStr=boolean
  Compare To Constant1 : simulink/Logic and Bit Operations/Compare To Constant  relop===  const=49  OutDataTypeStr=boolean
  Compare To Constant2 : simulink/Logic and Bit Operations/Compare To Constant  relop===  const=51  OutDataTypeStr=boolean
  Compare To Constant3 : simulink/Logic and Bit Operations/Compare To Constant  relop===  const=55  OutDataTypeStr=boolean
  Compare To Constant4 : simulink/Logic and Bit Operations/Compare To Constant  relop===  const=536  OutDataTypeStr=boolean
  Compare To Zero : simulink/Logic and Bit Operations/Compare To Zero  relop=~=  OutDataTypeStr=boolean
  Constant : Constant  Value=0  OutDataTypeStr=uint16
  Constant1 : Constant  Value=128  OutDataTypeStr=uint16
  Constant2 : Constant  Value=6  OutDataTypeStr=uint16
  Constant3 : Constant  Value=7  OutDataTypeStr=uint16
  Constant4 : Constant  Value=15  OutDataTypeStr=uint16
  Constant5 : Constant  Value=15  OutDataTypeStr=uint16
  Constant6 : Constant  Value=128  OutDataTypeStr=uint16
  Switch{,1..5} (6 alike) : Switch  Criteria=u2 > Threshold
  Control : Outport
  wires:
  Status/1 -> Compare To Constant4/1, Bitwise Operator/1, Bitwise Operator1/1
  Bitwise Operator1/1 -> Compare To Zero/1
  Compare To Zero/1 -> Switch/2
  Constant1/1 -> Switch/1
  Constant/1 -> Switch/3
  Compare To Constant/1 -> Switch1/2
  Switch/1 -> Switch1/3
  Bitwise Operator/1 -> Compare To Constant3/1, Compare To Constant2/1, Compare To Constant1/1, Compare To Constant/1
  Constant2/1 -> Switch1/1
  Compare To Constant1/1 -> Switch2/2
  Switch1/1 -> Switch2/3
  Constant3/1 -> Switch2/1
  Compare To Constant2/1 -> Switch3/2
  Switch2/1 -> Switch3/3
  Constant4/1 -> Switch3/1
  Compare To Constant3/1 -> Switch4/2
  Switch3/1 -> Switch4/3
  Constant5/1 -> Switch4/1
  Switch4/1 -> Switch5/3
  Compare To Constant4/1 -> Switch5/2
  Switch5/1 -> Control/1
  Constant6/1 -> Switch5/1

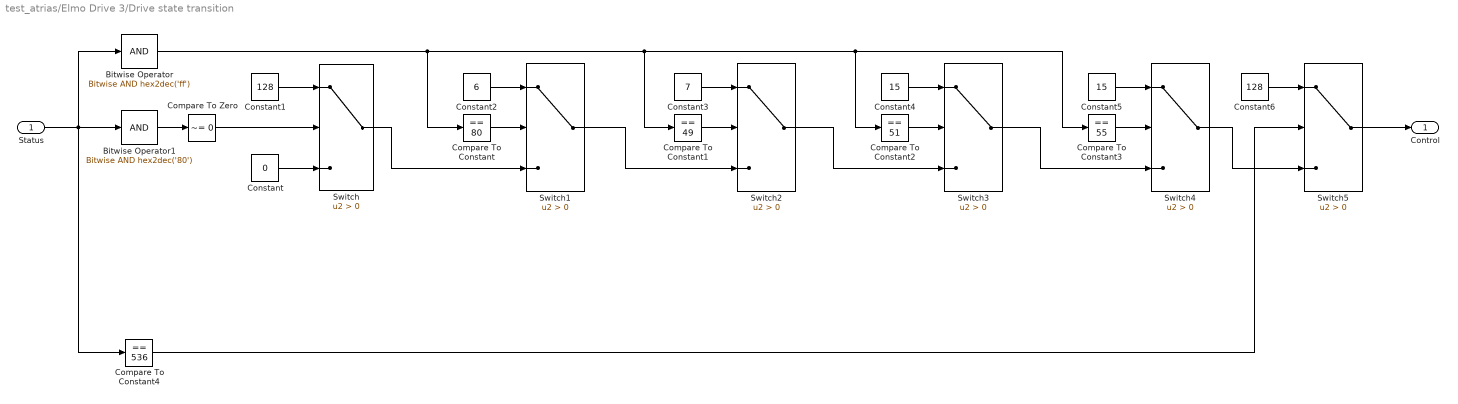
== system test_atrias/Elmo Drive 3/Drive state transition ==
  Status : Inport
  Bitwise Operator : simulink/Logic and Bit Operations/Bitwise Operator  logicop=AND  UseBitMask=on  BitMask=hex2dec('ff')  BitMaskRealWorld=Stored Integer
  Bitwise Operator1 : simulink/Logic and Bit Operations/Bitwise Operator  logicop=AND  UseBitMask=on  BitMask=hex2dec('80')  BitMaskRealWorld=Stored Integer
  Compare To Constant : simulink/Logic and Bit Operations/Compare To Constant  relop===  const=80  OutDataTypeStr=boolean
  Compare To Constant1 : simulink/Logic and Bit Operations/Compare To Constant  relop===  const=49  OutDataTypeStr=boolean
  Compare To Constant2 : simulink/Logic and Bit Operations/Compare To Constant  relop===  const=51  OutDataTypeStr=boolean
  Compare To Constant3 : simulink/Logic and Bit Operations/Compare To Constant  relop===  const=55  OutDataTypeStr=boolean
  Compare To Constant4 : simulink/Logic and Bit Operations/Compare To Constant  relop===  const=536  OutDataTypeStr=boolean
  Compare To Zero : simulink/Logic and Bit Operations/Compare To Zero  relop=~=  OutDataTypeStr=boolean
  Constant : Constant  Value=0  OutDataTypeStr=uint16
  Constant1 : Constant  Value=128  OutDataTypeStr=uint16
  Constant2 : Constant  Value=6  OutDataTypeStr=uint16
  Constant3 : Constant  Value=7  OutDataTypeStr=uint16
  Constant4 : Constant  Value=15  OutDataTypeStr=uint16
  Constant5 : Constant  Value=15  OutDataTypeStr=uint16
  Constant6 : Constant  Value=128  OutDataTypeStr=uint16
  Switch{,1..5} (6 alike) : Switch  Criteria=u2 > Threshold
  Control : Outport
  wires:
  Status/1 -> Compare To Constant4/1, Bitwise Operator/1, Bitwise Operator1/1
  Bitwise Operator1/1 -> Compare To Zero/1
  Compare To Zero/1 -> Switch/2
  Constant1/1 -> Switch/1
  Constant/1 -> Switch/3
  Compare To Constant/1 -> Switch1/2
  Switch/1 -> Switch1/3
  Bitwise Operator/1 -> Compare To Constant3/1, Compare To Constant2/1, Compare To Constant1/1, Compare To Constant/1
  Constant2/1 -> Switch1/1
  Compare To Constant1/1 -> Switch2/2
  Switch1/1 -> Switch2/3
  Constant3/1 -> Switch2/1
  Compare To Constant2/1 -> Switch3/2
  Switch2/1 -> Switch3/3
  Constant4/1 -> Switch3/1
  Compare To Constant3/1 -> Switch4/2
  Switch3/1 -> Switch4/3
  Constant5/1 -> Switch4/1
  Switch4/1 -> Switch5/3
  Compare To Constant4/1 -> Switch5/2
  Switch5/1 -> Control/1
  Constant6/1 -> Switch5/1

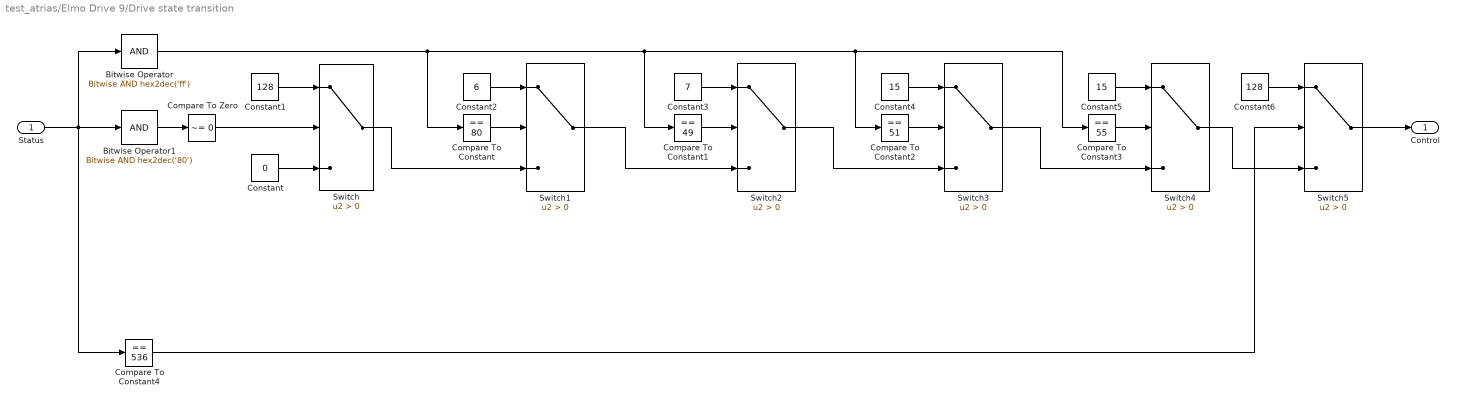
== system test_atrias/Elmo Drive 9/Drive state transition ==
  Status : Inport
  Bitwise Operator : simulink/Logic and Bit Operations/Bitwise Operator  logicop=AND  UseBitMask=on  BitMask=hex2dec('ff')  BitMaskRealWorld=Stored Integer
  Bitwise Operator1 : simulink/Logic and Bit Operations/Bitwise Operator  logicop=AND  UseBitMask=on  BitMask=hex2dec('80')  BitMaskRealWorld=Stored Integer
  Compare To Constant : simulink/Logic and Bit Operations/Compare To Constant  relop===  const=80  OutDataTypeStr=boolean
  Compare To Constant1 : simulink/Logic and Bit Operations/Compare To Constant  relop===  const=49  OutDataTypeStr=boolean
  Compare To Constant2 : simulink/Logic and Bit Operations/Compare To Constant  relop===  const=51  OutDataTypeStr=boolean
  Compare To Constant3 : simulink/Logic and Bit Operations/Compare To Constant  relop===  const=55  OutDataTypeStr=boolean
  Compare To Constant4 : simulink/Logic and Bit Operations/Compare To Constant  relop===  const=536  OutDataTypeStr=boolean
  Compare To Zero : simulink/Logic and Bit Operations/Compare To Zero  relop=~=  OutDataTypeStr=boolean
  Constant : Constant  Value=0  OutDataTypeStr=uint16
  Constant1 : Constant  Value=128  OutDataTypeStr=uint16
  Constant2 : Constant  Value=6  OutDataTypeStr=uint16
  Constant3 : Constant  Value=7  OutDataTypeStr=uint16
  Constant4 : Constant  Value=15  OutDataTypeStr=uint16
  Constant5 : Constant  Value=15  OutDataTypeStr=uint16
  Constant6 : Constant  Value=128  OutDataTypeStr=uint16
  Switch{,1..5} (6 alike) : Switch  Criteria=u2 > Threshold
  Control : Outport
  wires:
  Constant6/1 -> Switch5/1
  Switch5/1 -> Control/1
  Compare To Constant4/1 -> Switch5/2
  Switch4/1 -> Switch5/3
  Constant5/1 -> Switch4/1
  Switch3/1 -> Switch4/3
  Compare To Constant3/1 -> Switch4/2
  Constant4/1 -> Switch3/1
  Switch2/1 -> Switch3/3
  Compare To Constant2/1 -> Switch3/2
  Constant3/1 -> Switch2/1
  Switch1/1 -> Switch2/3
  Compare To Constant1/1 -> Switch2/2
  Constant2/1 -> Switch1/1
  Bitwise Operator/1 -> Compare To Constant/1, Compare To Constant1/1, Compare To Constant2/1, Compare To Constant3/1
  Switch/1 -> Switch1/3
  Compare To Constant/1 -> Switch1/2
  Constant/1 -> Switch/3
  Constant1/1 -> Switch/1
  Compare To Zero/1 -> Switch/2
  Bitwise Operator1/1 -> Compare To Zero/1
  Status/1 -> Bitwise Operator1/1, Bitwise Operator/1, Compare To Constant4/1
